simulink model "hbf_fft"  (R2015a)
settings: Solver=ode45  StartTime=0.0  StopTime=240300  RelTol=1e-3
model workspace (MAT data in the model file):
  AD_BP = Simulink.Parameter
  AD_BP.Value = 13
  AD_BP.DataType = 'auto'
  AD_W = Simulink.Parameter
  AD_W.Value = 14
  AD_W.DataType = 'auto'
undefined symbols (not defined in the file or in its folder): a, b
libraries: xbsIndex_r4 x234, dspswit3 x1, commanapbnd3 x1, commseqgen2 x1, dspsigops x1
(part 1 of 2)
settings Model: Creator=scott rogers  LastModifiedBy=scott rogers

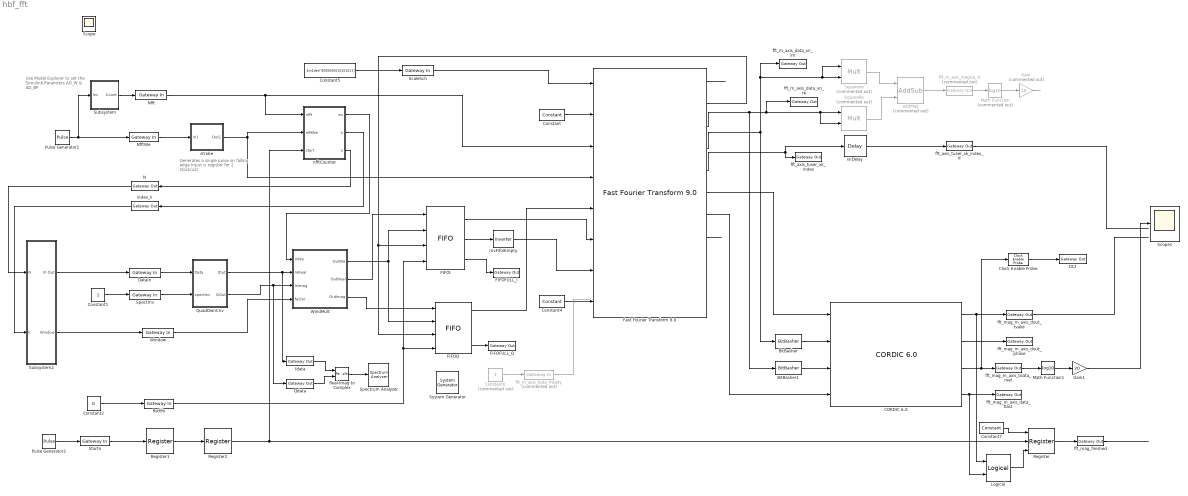
== system hbf_fft ==
  note: Generates a single pulse
      | on falling edge
      | Input is register for 2 Clock(x2)
  note: Use Model Explorer
      | to set the
      | Simulink.Paramters
      | AD_W &  AD_BP
  " System Generator" : xbsIndex_r4/ System Generator  Tag=genX  xilinxfamily=kintex7  part=xc7k160t  speed=-3  package=fbg676  synthesis_tool=Vivado  clock_wrapper=Clock Enables  directory=./netlist  proj_type=Vivado  Synth_file=Vivado Synthesis Defaults  Impl_file=Vivado Implementation Defaults  testbench=off  simulink_period=1  sysclk_period=10  dcm_input_clock_period=10  incr_netlist=off  trim_vbits=Everywhere in SubSystem  dbl_ovrd=According to Block Masks  core_generation=According to Block Masks  run_coregen=off  deprecated_control=off  eval_field=0  block_type=sysgen
  BitBasher : xbsIndex_r4/BitBasher  bitexpr=a={b[15],b[15:0]}  display_expr=off  sr_1=a  arith_type1="Signed  (2's comp)"  bin_pt1=15  sr_2=2  arith_type2=Unsigned  bin_pt2=0  sr_3=3  arith_type3=Unsigned  bin_pt3=0  sr_4=4  arith_type4=Unsigned  bin_pt4=0  dbl_ovrd=off  block_type=bitbasher
  BitBasher1 : xbsIndex_r4/BitBasher  bitexpr=a={b[15],b[15:0]}  display_expr=off  sr_1=a  arith_type1="Signed  (2's comp)"  bin_pt1=15  sr_2=2  arith_type2=Unsigned  bin_pt2=0  sr_3=3  arith_type3=Unsigned  bin_pt3=0  sr_4=4  arith_type4=Unsigned  bin_pt4=0  dbl_ovrd=off  block_type=bitbasher
  CE2 : xbsIndex_r4/Gateway Out  inherit_from_input=off  hdl_port=on  rows=1  columns=1  UseAsDAC=off  DACChannel='1'  interface=None  automatic_assignment=on  address_offset=hex2dec('00')  intf_name=''  intf_description=''  timing_constraint=None  locs_specified=off  LOCs={}  io_standard={}  block_type=gatewayout
  "CORDIC 6.0 " : xbsIndex_r4/CORDIC 6.0   functional_selection=Translate  architectural_configuration=Parallel  pipelining_mode=Maximum  data_format=UnsignedInteger  phase_format=Scaled_Radians  input_width=17  output_width=16  round_mode=Truncate  iterations=0  precision=0  compensation_scaling=No_Scale_Compensation  coarse_rotation=on  aclken=off  aresetn=off  out_tready=off  cartesian_has_tuser=off  cartesian_has_tlast=on  cartesian_tuser_width=1  phase_has_tuser=off  phase_has_tlast=off  phase_tuser_width=1  out_tlast_behv=Null  flow_control=NonBlocking  optimize_goal=Resources  trim_axipin_name=off  simulation_type=hybrid_sim  simulation_model=sysgen:cordic_v6_0  data_path_portlist={'s_axis_cartesian_tdata_imag', 's_axis_cartesian_tdata_real', 's_axis_phase_tdata_phase', 'm_axis_dout_tdata_imag', 'm_axis_dout_tdata_real', 'm_axis_dout_tdata_phase','m_axis_dout_tdata'}  ip_name=CORDIC  ip_version=6.0  dsptool_ready=true  ipcore_usecache=true  ipcore_useipmodelcache=true  wrapper_available=true  port_translation_map={ 'aclken' => 'en', 'aresetn' => 'rst' }  block_type=cordic_v6_0
      settings: infoedit=CORDIC 6.0
  Clock Enable Probe : xbsIndex_r4/Clock Enable Probe  inherit_constraints=on  block_type=ceprobe
      settings: infoedit="Clock enable extractor.  Produces a Boolean output that mirrors the hardware clock enable associated with the input sample rate.<br><br>Hardware notes: in hardware this block costs nothing."
  Constant : xbsIndex_r4/Constant  const=1.0  gui_display_data_type=Fixed-point  arith_type=Unsigned  n_bits=1  bin_pt=0  preci_type=Single  exp_width=8  frac_width=24  explicit_period=off  period=1  equ=P=C  opselect=C  inp2=PCIN>>17  opr=+  inp1=P  carry=CIN  dbl_ovrd=off  block_type=constant
  Constant1 : Constant
  Constant2 : Constant  Value=0
  Constant4 : xbsIndex_r4/Constant  const=0  gui_display_data_type=Boolean  arith_type=Boolean  n_bits=16  bin_pt=14  preci_type=Single  exp_width=8  frac_width=24  explicit_period=off  period=1  equ=P=C  opselect=C  inp2=PCIN>>17  opr=+  inp1=P  carry=CIN  dbl_ovrd=off  block_type=constant
  Constant5 : Constant  Value=bin2dec('0000000010101011')
  Constant6 : Constant  Commented=on
  Constant7 : xbsIndex_r4/Constant  const=1.0  gui_display_data_type=Boolean  arith_type=Boolean  n_bits=1  bin_pt=0  preci_type=Single  exp_width=8  frac_width=24  explicit_period=off  period=1  equ=P=C  opselect=C  inp2=PCIN>>17  opr=+  inp1=P  carry=CIN  dbl_ovrd=off  block_type=constant
  DataIn : xbsIndex_r4/Gateway In  gui_display_data_type=Fixed-point  arith_type="Signed  (2's comp)"  n_bits=AD_W  bin_pt=AD_BP  preci_type=Single  exp_width=8  frac_width=24  rows=1  columns=1  quantization="Round  (unbiased: +/- Inf)"  overflow=Saturate  period=1  UseAsADC=off  ADCChannel='1'  interface=None  automatic_assignment=on  address_offset=hex2dec('00')  intf_name=''  intf_description=''  timing_constraint=None  locs_specified=off  LOCs={}  io_standard={}  inherit_from_input=off  hdl_port=on  dbl_ovrd=off  block_type=gatewayin
  FIFOFULL_I : xbsIndex_r4/Gateway Out  inherit_from_input=off  hdl_port=on  rows=1  columns=1  UseAsDAC=off  DACChannel='1'  interface=None  automatic_assignment=on  address_offset=hex2dec('00')  intf_name=''  intf_description=''  timing_constraint=None  locs_specified=off  LOCs={}  io_standard={}  block_type=gatewayout
  FIFOFULL_Q : xbsIndex_r4/Gateway Out  inherit_from_input=off  hdl_port=on  rows=1  columns=1  UseAsDAC=off  DACChannel='1'  interface=None  automatic_assignment=on  address_offset=hex2dec('00')  intf_name=''  intf_description=''  timing_constraint=None  locs_specified=off  LOCs={}  io_standard={}  block_type=gatewayout
  FIFOI : xbsIndex_r4/FIFO  mem_type=Block RAM  performance_options=Standard_FIFO  embedded_registers=off  depth=16  percent_nbits=2  rst=on  rst_latency=1  en=off  use_dcount=off  use_percent_full_port=off  use_almost_empty=off  almost_empty_thresh=2  use_almost_full=off  almost_full_thresh=14  explicit_period=off  dbl_ovrd=off  block_type=fifo
  FIFOQ : xbsIndex_r4/FIFO  mem_type=Block RAM  performance_options=Standard_FIFO  embedded_registers=off  depth=16  percent_nbits=1  rst=on  rst_latency=1  en=off  use_dcount=off  use_percent_full_port=off  use_almost_empty=off  almost_empty_thresh=2  use_almost_full=off  almost_full_thresh=14  explicit_period=off  dbl_ovrd=off  block_type=fifo
  "Fast Fourier Transform 9.0 " : xbsIndex_r4/Fast Fourier Transform 9.0   transform_length=4096  target_clock_frequency=93  target_data_throughput=50  implementation_options=radix_4_burst_io  run_time_configurable_transform_length=on  phase_factor_width=32  scaling_options=scaled  rounding_modes=truncation  aclken=off  aresetn=off  cyclic_prefix_insertion=off  output_ordering=natural_order  throttle_scheme=realtime  xk_index=on  ovflo=off  trim_axipin_name=off  memory_options_data=block_ram  memory_options_phase_factors=block_ram  number_of_stages_using_block_ram_for_data_and_phase_factors=1  memory_options_reorder=block_ram  memory_options_hybrid=off  complex_mult_type=use_mults_resources  butterfly_type=use_luts  simulation_type=hybrid_sim  simulation_model=sysgen:xfftv9_cmodel  data_path_portlist={ 's_axis_data_tdata', 'm_axis_data_tdata', 'm_axis_status_tdata', 'event_fft_overflow' }  channels=1  input_ordering=natural_order  input_width=16  ip_name=Fast Fourier Transform  ip_version=9.0  dsptool_ready=true  ipcore_usecache=true  ipcore_useipmodelcache=true  wrapper_available=true  port_translation_map={ 'aclken' => 'en', 'aresetn' => 'rst'}  data_format=fixed_point  block_type=xfft_v9_0
  Gain : Gain  Commented=on  Gain=10
  Gain1 : Gain  Gain=20
  Idata : xbsIndex_r4/Gateway Out  inherit_from_input=off  hdl_port=on  rows=1  columns=1  UseAsDAC=off  DACChannel='1'  interface=None  automatic_assignment=on  address_offset=hex2dec('00')  intf_name=''  intf_description=''  timing_constraint=None  locs_specified=off  LOCs={}  io_standard={}  block_type=gatewayout
  InvFifoIEmpty : xbsIndex_r4/Inverter  en=off  latency=0  dbl_ovrd=off  block_type=inv
  Logical : xbsIndex_r4/Logical  logical_function=AND  inputs=2  en=off  latency=1  precision=Full  arith_type=Unsigned  n_bits=16  bin_pt=0  align_bp=on  dbl_ovrd=off  block_type=logical
  Math Function : Math  Commented=on  Operator=log10  SaturateOnIntegerOverflow=on
  Math Function1 : Math  Operator=log10  SaturateOnIntegerOverflow=on
  N : xbsIndex_r4/Gateway Out  inherit_from_input=off  hdl_port=on  rows=1  columns=1  UseAsDAC=off  DACChannel='1'  interface=None  automatic_assignment=on  address_offset=hex2dec('00')  intf_name=''  intf_description=''  timing_constraint=None  locs_specified=off  LOCs={}  io_standard={}  block_type=gatewayout
  Nfft : xbsIndex_r4/Gateway In  gui_display_data_type=Fixed-point  arith_type=Unsigned  n_bits=5  bin_pt=0  preci_type=Single  exp_width=8  frac_width=24  rows=1  columns=1  quantization="Round  (unbiased: +/- Inf)"  overflow=Wrap  period=2  UseAsADC=off  ADCChannel='1'  interface=None  automatic_assignment=on  address_offset=hex2dec('00')  intf_name=''  intf_description=''  timing_constraint=None  locs_specified=off  LOCs={}  io_standard={}  inherit_from_input=off  hdl_port=on  dbl_ovrd=off  block_type=gatewayin
  NfftWe : xbsIndex_r4/Gateway In  gui_display_data_type=Boolean  arith_type=Boolean  n_bits=16  bin_pt=14  preci_type=Single  exp_width=8  frac_width=24  rows=1  columns=1  quantization="Round  (unbiased: +/- Inf)"  overflow=Saturate  period=2  UseAsADC=off  ADCChannel='1'  interface=None  automatic_assignment=on  address_offset=hex2dec('00')  intf_name=''  intf_description=''  timing_constraint=None  locs_specified=off  LOCs={}  io_standard={}  inherit_from_input=off  hdl_port=on  dbl_ovrd=off  block_type=gatewayin
  Pulse Generator1 : DiscretePulseGenerator  Period=30000  PulseWidth=8  PhaseDelay=10
  Pulse Generator2 : DiscretePulseGenerator  Period=30000  PulseWidth=21  PhaseDelay=38
  Qdata : xbsIndex_r4/Gateway Out  inherit_from_input=off  hdl_port=on  rows=1  columns=1  UseAsDAC=off  DACChannel='1'  interface=None  automatic_assignment=on  address_offset=hex2dec('00')  intf_name=''  intf_description=''  timing_constraint=None  locs_specified=off  LOCs={}  io_standard={}  block_type=gatewayout
  QuadDwnCnv : Subsystem
  Real-Imag to Complex : RealImagToComplex
  Register : xbsIndex_r4/Register  init=0  rst=on  en=on  dbl_ovrd=off  block_type=register
  Register1 : xbsIndex_r4/Register  init=0  rst=off  en=off  dbl_ovrd=off  block_type=register
  Register2 : xbsIndex_r4/Register  init=0  rst=off  en=off  dbl_ovrd=off  block_type=register
  Rstfifo : xbsIndex_r4/Gateway In  gui_display_data_type=Boolean  arith_type=Boolean  n_bits=16  bin_pt=14  preci_type=Single  exp_width=8  frac_width=24  rows=1  columns=1  quantization="Round  (unbiased: +/- Inf)"  overflow=Saturate  period=2  UseAsADC=off  ADCChannel='1'  interface=None  automatic_assignment=on  address_offset=hex2dec('00')  intf_name=''  intf_description=''  timing_constraint=None  locs_specified=off  LOCs={}  io_standard={}  inherit_from_input=off  hdl_port=on  dbl_ovrd=off  block_type=gatewayin
  ScaleSch : xbsIndex_r4/Gateway In  gui_display_data_type=Fixed-point  arith_type=Unsigned  n_bits=12  bin_pt=0  preci_type=Single  exp_width=8  frac_width=24  rows=1  columns=1  quantization="Round  (unbiased: +/- Inf)"  overflow=Wrap  period=2  UseAsADC=off  ADCChannel='1'  interface=None  automatic_assignment=on  address_offset=hex2dec('00')  intf_name=''  intf_description=''  timing_constraint=None  locs_specified=off  LOCs={}  io_standard={}  inherit_from_input=off  hdl_port=on  dbl_ovrd=off  block_type=gatewayin
  Scope1 : Scope
      settings: TimeRange=200000  YMin=-51.8234  YMax=-51.8234  MaxDataPoints=15000
  SpectInv : xbsIndex_r4/Gateway In  gui_display_data_type=Fixed-point  arith_type=Unsigned  n_bits=1  bin_pt=0  preci_type=Single  exp_width=8  frac_width=24  rows=1  columns=1  quantization="Round  (unbiased: +/- Inf)"  overflow=Wrap  period=2  UseAsADC=off  ADCChannel='1'  interface=None  automatic_assignment=on  address_offset=hex2dec('00')  intf_name=''  intf_description=''  timing_constraint=None  locs_specified=off  LOCs={}  io_standard={}  inherit_from_input=off  hdl_port=on  dbl_ovrd=off  block_type=gatewayin
  Spectrum Analyzer : SpectrumAnalyzer
  SquareIm : xbsIndex_r4/Mult  Commented=on  precision=Full  arith_type="Signed  (2's comp)"  n_bits=17  bin_pt=15  quantization=Truncate  overflow=Wrap  en=off  latency=3  use_behavioral_HDL=off  opt=Speed  use_embedded=on  optimum_pipeline=off  pipeline=on  dbl_ovrd=off  use_rpm=on  placement_style=Triangular  block_type=mult
  SquareRe : xbsIndex_r4/Mult  Commented=on  precision=Full  arith_type="Signed  (2's comp)"  n_bits=17  bin_pt=15  quantization=Truncate  overflow=Wrap  en=off  latency=3  use_behavioral_HDL=off  opt=Speed  use_embedded=on  optimum_pipeline=off  pipeline=on  dbl_ovrd=off  use_rpm=on  placement_style=Triangular  block_type=mult
  Startn : xbsIndex_r4/Gateway In  gui_display_data_type=Boolean  arith_type=Boolean  n_bits=16  bin_pt=14  preci_type=Single  exp_width=8  frac_width=24  rows=1  columns=1  quantization="Round  (unbiased: +/- Inf)"  overflow=Saturate  period=2  UseAsADC=off  ADCChannel='1'  interface=None  automatic_assignment=on  address_offset=hex2dec('00')  intf_name=''  intf_description=''  timing_constraint=None  locs_specified=off  LOCs={}  io_standard={}  inherit_from_input=off  hdl_port=on  dbl_ovrd=off  block_type=gatewayin
  Subsystem : Subsystem
  Subsystem2 : Subsystem
  WindMult : Subsystem
  Window : xbsIndex_r4/Gateway In  gui_display_data_type=Fixed-point  arith_type=Unsigned  n_bits=16  bin_pt=14  preci_type=Single  exp_width=8  frac_width=24  rows=1  columns=1  quantization="Round  (unbiased: +/- Inf)"  overflow=Wrap  period=2  UseAsADC=off  ADCChannel='1'  interface=None  automatic_assignment=on  address_offset=hex2dec('00')  intf_name=''  intf_description=''  timing_constraint=None  locs_specified=off  LOCs={}  io_standard={}  inherit_from_input=off  hdl_port=on  dbl_ovrd=off  block_type=gatewayin
  addMag : xbsIndex_r4/AddSub  Commented=on  mode=Addition  use_carryin=off  use_carryout=off  en=off  latency=1  precision=Full  arith_type=Unsigned  n_bits=16  bin_pt=14  quantization=Truncate  overflow=Wrap  use_behavioral_HDL=off  hw_selection=Fabric  pipelined=off  dbl_ovrd=off  block_type=addsub
  fft_axis_tuser_xk_index : xbsIndex_r4/Gateway Out  inherit_from_input=off  hdl_port=off  rows=1  columns=1  UseAsDAC=off  DACChannel='1'  interface=None  automatic_assignment=on  address_offset=hex2dec('00')  intf_name=''  intf_description=''  timing_constraint=None  locs_specified=off  LOCs={}  io_standard={}  block_type=gatewayout
  fft_axis_tuser_xk_index_d : xbsIndex_r4/Gateway Out  inherit_from_input=off  hdl_port=on  rows=1  columns=1  UseAsDAC=off  DACChannel='1'  interface=None  automatic_assignment=on  address_offset=hex2dec('00')  intf_name=''  intf_description=''  timing_constraint=None  locs_specified=off  LOCs={}  io_standard={}  block_type=gatewayout
  fft_m_axis_data_tready : xbsIndex_r4/Gateway In  Commented=on  gui_display_data_type=Boolean  arith_type=Boolean  n_bits=16  bin_pt=14  preci_type=Single  exp_width=8  frac_width=24  rows=1  columns=1  quantization="Round  (unbiased: +/- Inf)"  overflow=Saturate  period=2  UseAsADC=off  ADCChannel='1'  interface=None  automatic_assignment=on  address_offset=hex2dec('00')  intf_name=''  intf_description=''  timing_constraint=None  locs_specified=off  LOCs={}  io_standard={}  inherit_from_input=off  hdl_port=on  dbl_ovrd=off  block_type=gatewayin
  fft_m_axis_data_xn_im : xbsIndex_r4/Gateway Out  inherit_from_input=off  hdl_port=off  rows=1  columns=1  UseAsDAC=off  DACChannel='1'  interface=None  automatic_assignment=on  address_offset=hex2dec('00')  intf_name=''  intf_description=''  timing_constraint=None  locs_specified=off  LOCs={}  io_standard={}  block_type=gatewayout
  fft_m_axis_data_xn_re : xbsIndex_r4/Gateway Out  inherit_from_input=off  hdl_port=off  rows=1  columns=1  UseAsDAC=off  DACChannel='1'  interface=None  automatic_assignment=on  address_offset=hex2dec('00')  intf_name=''  intf_description=''  timing_constraint=None  locs_specified=off  LOCs={}  io_standard={}  block_type=gatewayout
  fft_m_axis_magSq_d : xbsIndex_r4/Gateway Out  Commented=on  inherit_from_input=off  hdl_port=on  rows=1  columns=1  UseAsDAC=off  DACChannel='1'  interface=None  automatic_assignment=on  address_offset=hex2dec('00')  intf_name=''  intf_description=''  timing_constraint=None  locs_specified=off  LOCs={}  io_standard={}  block_type=gatewayout
  fft_mag_finished : xbsIndex_r4/Gateway Out  inherit_from_input=off  hdl_port=on  rows=1  columns=1  UseAsDAC=off  DACChannel='1'  interface=None  automatic_assignment=on  address_offset=hex2dec('00')  intf_name=''  intf_description=''  timing_constraint=None  locs_specified=off  LOCs={}  io_standard={}  block_type=gatewayout
  fft_mag_m_axis_data_tlast : xbsIndex_r4/Gateway Out  inherit_from_input=off  hdl_port=on  rows=1  columns=1  UseAsDAC=off  DACChannel='1'  interface=None  automatic_assignment=on  address_offset=hex2dec('00')  intf_name=''  intf_description=''  timing_constraint=None  locs_specified=off  LOCs={}  io_standard={}  block_type=gatewayout
  fft_mag_m_axis_dout_phase : xbsIndex_r4/Gateway Out  inherit_from_input=off  hdl_port=off  rows=1  columns=1  UseAsDAC=off  DACChannel='1'  interface=None  automatic_assignment=on  address_offset=hex2dec('00')  intf_name=''  intf_description=''  timing_constraint=None  locs_specified=off  LOCs={}  io_standard={}  block_type=gatewayout
  fft_mag_m_axis_dout_tvalid : xbsIndex_r4/Gateway Out  inherit_from_input=off  hdl_port=on  rows=1  columns=1  UseAsDAC=off  DACChannel='1'  interface=None  automatic_assignment=on  address_offset=hex2dec('00')  intf_name=''  intf_description=''  timing_constraint=None  locs_specified=off  LOCs={}  io_standard={}  block_type=gatewayout
  fft_mag_m_axis_tdata_real : xbsIndex_r4/Gateway Out  inherit_from_input=off  hdl_port=on  rows=1  columns=1  UseAsDAC=off  DACChannel='1'  interface=None  automatic_assignment=on  address_offset=hex2dec('00')  intf_name=''  intf_description=''  timing_constraint=None  locs_specified=off  LOCs={}  io_standard={}  block_type=gatewayout
  index_k : xbsIndex_r4/Gateway Out  inherit_from_input=off  hdl_port=on  rows=1  columns=1  UseAsDAC=off  DACChannel='1'  interface=None  automatic_assignment=on  address_offset=hex2dec('00')  intf_name=''  intf_description=''  timing_constraint=None  locs_specified=off  LOCs={}  io_standard={}  block_type=gatewayout
  nfftCounter : Subsystem
  strobe : Subsystem
  xnDelay : xbsIndex_r4/Delay  rst=off  infoeditControl=Selection of Reset will increase slice count due to use of real FFs and instead of SRLs  en=off  latency=20  reg_retiming=on  dbl_ovrd=off  block_type=delay
  Scope : Scope
  wires:
  FIFOI/2 -> InvFifoIEmpty/1
  InvFifoIEmpty/1 -> "Fast Fourier Transform 9.0 "/7
  FIFOI/1 -> "Fast Fourier Transform 9.0 "/6
  FIFOQ/1 -> "Fast Fourier Transform 9.0 "/5
  Nfft/1 -> "Fast Fourier Transform 9.0 "/3, nfftCounter/1(nfft)
  Constant/1 -> "Fast Fourier Transform 9.0 "/2
  Startn/1 -> Register1/1
  "Fast Fourier Transform 9.0 "/5 -> fft_axis_tuser_xk_index/1, xnDelay/1
  "Fast Fourier Transform 9.0 "/4 -> BitBasher/1, SquareIm/2, SquareIm/1, fft_m_axis_data_xn_im/1
  Pulse Generator2/1 -> Startn/1
  "Fast Fourier Transform 9.0 "/2 -> FIFOQ/3, FIFOI/3
  FIFOQ/3 -> FIFOFULL_Q/1
  FIFOI/3 -> FIFOFULL_I/1
  Constant4/1 -> "Fast Fourier Transform 9.0 "/8
  nfftCounter/1(en) -> WindMult/1(InWe)
  DataIn/1 -> QuadDwnCnv/1(Data)
  SquareIm/1 -> addMag/1
  SquareRe/1 -> addMag/2
  Pulse Generator1/1 -> NfftWe/1, Subsystem/1(Inc)
  Idata/1 -> Real-Imag to Complex/1
  Qdata/1 -> Real-Imag to Complex/2
  addMag/1 -> fft_m_axis_magSq_d/1
  SpectInv/1 -> QuadDwnCnv/2(spectInv)
  Constant1/1 -> SpectInv/1
  fft_m_axis_magSq_d/1 -> Math Function/1
  Math Function/1 -> Gain/1
  Gain/1 -> ?
  xnDelay/1 -> fft_axis_tuser_xk_index_d/1
  Constant2/1 -> Rstfifo/1
  Rstfifo/1 -> FIFOQ/4, FIFOI/4
  Constant6/1 -> fft_m_axis_data_tready/1
  fft_mag_m_axis_tdata_real/1 -> Math Function1/1
  Math Function1/1 -> Gain1/1
  Gain1/1 -> Scope1/1
  BitBasher/1 -> "CORDIC 6.0 "/2
  BitBasher1/1 -> "CORDIC 6.0 "/3
  fft_mag_m_axis_dout_tvalid/1 -> ?
  "CORDIC 6.0 "/1 -> Logical/1, fft_mag_m_axis_dout_tvalid/1
  "CORDIC 6.0 "/4 -> Logical/2, fft_mag_m_axis_data_tlast/1
  "Fast Fourier Transform 9.0 "/7 -> "CORDIC 6.0 "/4
  fft_axis_tuser_xk_index_d/1 -> ?
  "CORDIC 6.0 "/2 -> fft_mag_m_axis_dout_phase/1
  Constant7/1 -> Register/1
  Register/1 -> fft_mag_finished/1
  fft_mag_finished/1 -> ?
  strobe/1(Out1) -> "Fast Fourier Transform 9.0 "/4, nfftCounter/2(nfftWe)
  QuadDwnCnv/2(QOut) -> Qdata/1, WindMult/3(InImag)
  QuadDwnCnv/1(IOut) -> Idata/1, WindMult/2(inReal)
  nfftCounter/2(k) -> index_k/1
  Window/1 -> WindMult/4(factor)
  WindMult/2(OutReal) -> FIFOI/1
  WindMult/3(OutImag) -> FIFOQ/1
  WindMult/1(OutWe) -> FIFOQ/2, FIFOI/2
  nfftCounter/3(n) -> N/1
  Register1/1 -> Register2/1
  "Fast Fourier Transform 9.0 "/3 -> BitBasher1/1, fft_m_axis_data_xn_re/1, SquareRe/2, SquareRe/1
  Register2/1 -> Register/2, nfftCounter/3(start)
  Subsystem/1(Count) -> Nfft/1
  NfftWe/1 -> strobe/1(In1)
  N/1 -> Subsystem2/1(N)
  index_k/1 -> Subsystem2/2(k)
  Subsystem2/1(IF Out) -> DataIn/1
  Subsystem2/2(Window) -> Window/1
  "Fast Fourier Transform 9.0 "/6 -> "CORDIC 6.0 "/1
  "CORDIC 6.0 "/3 -> Clock Enable Probe/1, fft_mag_m_axis_tdata_real/1
  fft_m_axis_data_tready/1 -> ?
  "Fast Fourier Transform 9.0 "/8 -> ?
  Real-Imag to Complex/1 -> Spectrum Analyzer/1
  ScaleSch/1 -> "Fast Fourier Transform 9.0 "/1
  Constant5/1 -> ScaleSch/1
  "Fast Fourier Transform 9.0 "/1 -> ?
  Logical/1 -> Register/3
  Clock Enable Probe/1 -> CE2/1

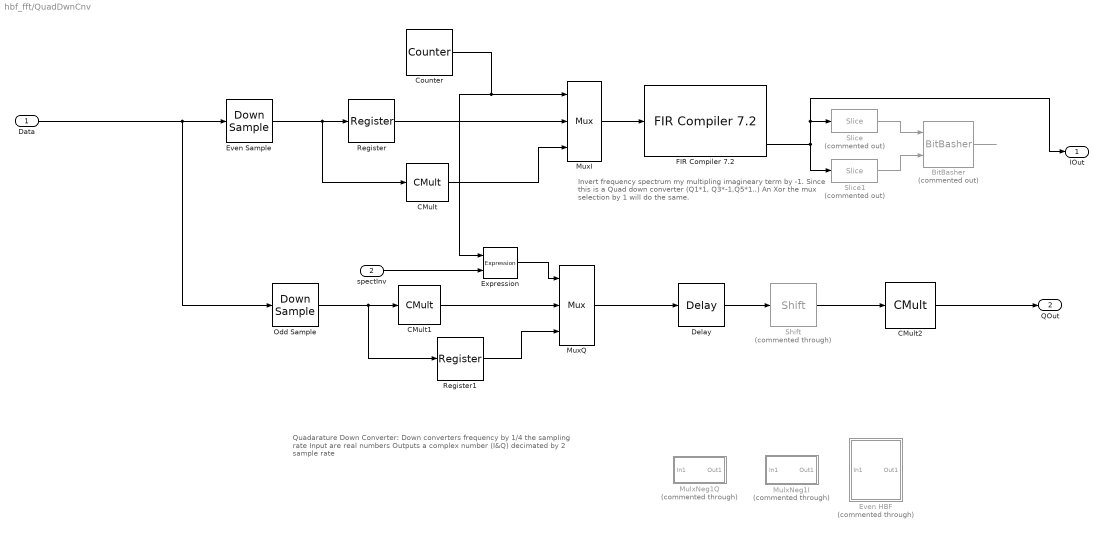
== system hbf_fft/QuadDwnCnv ==
  note: Invert frequency spectrum my multipling imagineary term by -1.
      | Since this is a Quad down converter (Q1*1, Q3*-1,Q5*1..)
      | An Xor the mux selection by 1 will do the same.
  note: Quadarature Down Converter:
      | Down converters frequency by 1/4 the sampling rate
      | Input are real numbers
      | Outputs a complex number (I&Q) decimated by 2 sample rate
  Data : Inport
  spectInv : Inport  Port=2
  BitBasher : xbsIndex_r4/BitBasher  Commented=on  bitexpr=a={b,c}  display_expr=off  sr_1=a  arith_type1="Signed  (2's comp)"  bin_pt1=13  sr_2=2  arith_type2=Unsigned  bin_pt2=0  sr_3=3  arith_type3=Unsigned  bin_pt3=0  sr_4=4  arith_type4=Unsigned  bin_pt4=0  dbl_ovrd=off  block_type=bitbasher
  CMult : xbsIndex_r4/CMult  const=-1  gui_display_data_type=Fixed-point  const_n_bits=14  const_bin_pt=13  float_type=Single  exp_bits=8  fraction_bits=24  en=off  latency=1  precision=User Defined  arith_type="Signed  (2's comp)"  n_bits=14  bin_pt=13  quantization=Truncate  overflow=Saturate  use_behavioral_HDL=off  mem_type=Distributed RAM  pipeline=off  dbl_ovrd=off  block_type=cmult
  CMult1 : xbsIndex_r4/CMult  const=-1  gui_display_data_type=Fixed-point  const_n_bits=14  const_bin_pt=13  float_type=Single  exp_bits=8  fraction_bits=24  en=off  latency=1  precision=User Defined  arith_type="Signed  (2's comp)"  n_bits=14  bin_pt=13  quantization=Truncate  overflow=Saturate  use_behavioral_HDL=off  mem_type=Distributed RAM  pipeline=off  dbl_ovrd=off  block_type=cmult
  CMult2 : xbsIndex_r4/CMult  const=.5  gui_display_data_type=Fixed-point  const_n_bits=16  const_bin_pt=14  float_type=Single  exp_bits=8  fraction_bits=24  en=off  latency=1  precision=User Defined  arith_type="Signed  (2's comp)"  n_bits=16  bin_pt=14  quantization=Truncate  overflow=Wrap  use_behavioral_HDL=off  mem_type=Distributed RAM  pipeline=off  dbl_ovrd=off  block_type=cmult
  Counter : xbsIndex_r4/Counter  cnt_type=Count Limited  cnt_to=1  operation=Up  start_count=0  cnt_by_val=1  arith_type=Unsigned  n_bits=1  bin_pt=0  load_pin=off  rst=off  en=off  explicit_period=on  period=2  use_behavioral_HDL=off  implementation=Fabric  dbl_ovrd=off  block_type=counter
  Delay : xbsIndex_r4/Delay  rst=off  infoeditControl=Selection of Reset will increase slice count due to use of real FFs and instead of SRLs  en=off  latency=17  reg_retiming=off  dbl_ovrd=off  block_type=delay
  Even HBF : Subsystem  Commented=through  mask{coe=|, numbits=16, binarypoint=16}
      mask coe=|
      | [5.78745247606902e-07	-6.34583335209700e-06	3.11100665493994e-05	-9.81618504431095e-05	0.000251198104263337	-0.000560678336657476	0.00113068456439032	-0.00210596116830266	0.00368000288358338	-0.00610797832934512	0.00973476334993138	-0.0150640153636479	0.0229388203755087	-0.0350608263163152	0.0557915831460557	-0.101197280248630	0.316642817526843
      | ]
      mask prompts: coe "Coefficent"; numbits "Number of Bits"; binarypoint "Binary Point"
  Even Sample : xbsIndex_r4/Down Sample  sample_ratio=2  sample_phase=First Value of Frame  en=off  rst=off  latency=1  dbl_ovrd=off  block_type=dsamp
  Expression : xbsIndex_r4/Expression  expression=a ^ b  align_bp=on  en=off  latency=0  precision=Full  arith_type=Unsigned  n_bits=16  bin_pt=0  dbl_ovrd=off  block_type=expr
  "FIR Compiler 7.2 " : xbsIndex_r4/FIR Compiler 7.2   coefficientvector=[0.00115083621567666,-0.00274368371137841,0.00575557363771786,-0.0107205402010719,0.0185625473110580,-0.0310523194554332,0.0525318906465399,-0.0990035964397264,0.315519291996618,0.315519291996618,-0.0990035964397264,0.0525318906465399,-0.0310523194554332,0.0185625473110580,-0.0107205402010719,0.00575557363771786,-0.00274368371137841,0.00115083621567666]  coefficient_sets=1  coefficient_reload=off  filter_type=Single_Rate  rate_change_type=Integer  interpolation_rate=1  decimation_rate=1  zero_pack_factor=1  channel_sequence=Basic  number_channels=1  pattern_list='P4-0,P4-1,P4-2,P4-3,P4-4'  number_paths=1  ratespecification=Maximum_Possible  sampleperiod=2  hardwareoversamplingrate=1  coefficient_sign=Signed  quantization=Quantize_Only  coefficient_width=16  bestprecision=on  coefficient_fractional_bits=16  coefficient_structure=Inferred  output_rounding_mode=Truncate_LSBs  output_width=19  filter_architecture=Systolic_Multiply_Accumulate  optimization_goal=Area  optimization_list='None'  data_buffer_type=Automatic  coefficient_buffer_type=Automatic  input_buffer_type=Automatic  output_buffer_type=Automatic  preference_for_other_storage=Automatic  multi_column_support=Automatic  columnconfig='9'  inter_column_pipe_length=4  data_has_tlast=Not_Required  m_data_has_tready=off  s_data_has_fifo=off  s_data_has_tuser=Not_Required  m_data_has_tuser=Not_Required  s_config_sync_mode=On_Vector  s_config_method=Single  num_reload_slots=1  has_aclken=off  has_aresetn=off  infoeditControl=ARESETn must be asserted for a minimum of 2 cycles  reset_data_vector=on  trim_axipin_name=on  simulation_type=hybrid_sim  simulation_model=sysgen:xfirv7_2_cmodel  data_path_portlist={ 's_axis_data_tdata', 'm_axis_data_tdata' }  passband_min=0.0  passband_max=0.5  stopband_min=0.5  stopband_max=1.0  filter_selection=1  gui_behaviour='Sysgen_GUI'  data_sign=Signed  data_width=16  data_fractional_bits=0  data_tuser_width=1  wrapper_available=true  ip_wrap_arbitrary_binary_point=true  ip_name=FIR Compiler  ip_version=7.2  dsptool_ready=true  ipcore_usecache=true  ipcore_useipmodelcache=true  port_translation_map={ 'aclken' => 'en', 'aresetn' => 'rst' }  run_core_at_system_period=true  ipcore_xco_need_fpga_part=true  block_type=fir_compiler_v7_2
      settings: infoedit=Maximum Possible : Maximizes oversampling rate. Abstracted input handshake (no s_data_tvalid) and automatic rate propagation.<br>Hardware Oversampling Rate : Specifies oversampling rate relative to the input sample period. Abstracted input handshake (no s_data_tvalid) and automatic rate propagation.<br>Input/Output Sample Period : Specifies absolute oversampling rate. No input handshake abstraction (exposes s_data_tvalid) and no rate propagation.
  MulxNeg1I : Subsystem  Commented=through
  MulxNeg1Q : Subsystem  Commented=through
  MuxI : xbsIndex_r4/Mux  inputs=2  en=off  latency=1  precision=Full  arith_type=Unsigned  n_bits=16  bin_pt=14  quantization=Truncate  overflow=Wrap  dbl_ovrd=off  block_type=mux
  MuxQ : xbsIndex_r4/Mux  inputs=2  en=off  latency=1  precision=Full  arith_type=Unsigned  n_bits=16  bin_pt=14  quantization=Truncate  overflow=Wrap  dbl_ovrd=off  block_type=mux
  Odd Sample : xbsIndex_r4/Down Sample  sample_ratio=2  sample_phase="Last Value of Frame  (most efficient)"  en=off  rst=off  latency=1  dbl_ovrd=off  block_type=dsamp
  Register : xbsIndex_r4/Register  init=0  rst=off  en=off  dbl_ovrd=off  block_type=register
  Register1 : xbsIndex_r4/Register  init=0  rst=off  en=off  dbl_ovrd=off  block_type=register
  Shift : xbsIndex_r4/Shift  Commented=through  shift_dir=Right  shift_bits=1  en=off  latency=1  precision=Full  arith_type="Signed  (2's comp)"  n_bits=15  bin_pt=14  quantization=Truncate  overflow=Wrap  dbl_ovrd=off  block_type=shift
  Slice : xbsIndex_r4/Slice  Commented=on  nbits=1  boolean_output=off  mode=Upper Bit Location + Width  bit1=0  base1=MSB of Input  bit0=-13  base0=Binary Point of Input  dbl_ovrd=off  block_type=slice
  Slice1 : xbsIndex_r4/Slice  Commented=on  nbits=13  boolean_output=off  mode=Two Bit Locations  bit1=-1  base1=Binary Point of Input  bit0=-13  base0=Binary Point of Input  dbl_ovrd=off  block_type=slice
  IOut : Outport
  QOut : Outport  Port=2
  wires:
  Even Sample/1 -> CMult/1, Register/1
  CMult1/1 -> MuxQ/2
  Counter/1 -> MuxI/1, Expression/1
  Odd Sample/1 -> CMult1/1, Register1/1
  Register/1 -> MuxI/2
  Register1/1 -> MuxQ/3
  Expression/1 -> MuxQ/1
  spectInv/1 -> Expression/2
  Data/1 -> Odd Sample/1, Even Sample/1
  Delay/1 -> Shift/1
  MuxI/1 -> "FIR Compiler 7.2 "/1
  MuxQ/1 -> Delay/1
  Shift/1 -> CMult2/1
  "FIR Compiler 7.2 "/3 -> Slice1/1, IOut/1, Slice/1
  Slice/1 -> BitBasher/1
  BitBasher/1 -> ?
  Slice1/1 -> BitBasher/2
  CMult/1 -> MuxI/3
  CMult2/1 -> QOut/1

== system hbf_fft/Subsystem ==
  Inc : Inport
  Constant : Constant  Value=10
  Counter : dspswit3/Counter  Direction=Up  CountEvent=Falling edge  CounterSize=User defined  MaxCount=1  InitialCount=0  Output=Count  HitValue=32  ResetInput=off  SamplesPerFrame=1  Ts=1  CntDtype=double  HitDtype=Logical
  Manual Switch : ManualSwitch  CurrentSetting=0
  Sum : Sum  Inputs=|++
  Count : Outport
  wires:
  Inc/1 -> Counter/1
  Counter/1 -> Sum/1
  Constant/1 -> Manual Switch/2, Sum/2
  Sum/1 -> Manual Switch/1
  Manual Switch/1 -> Count/1

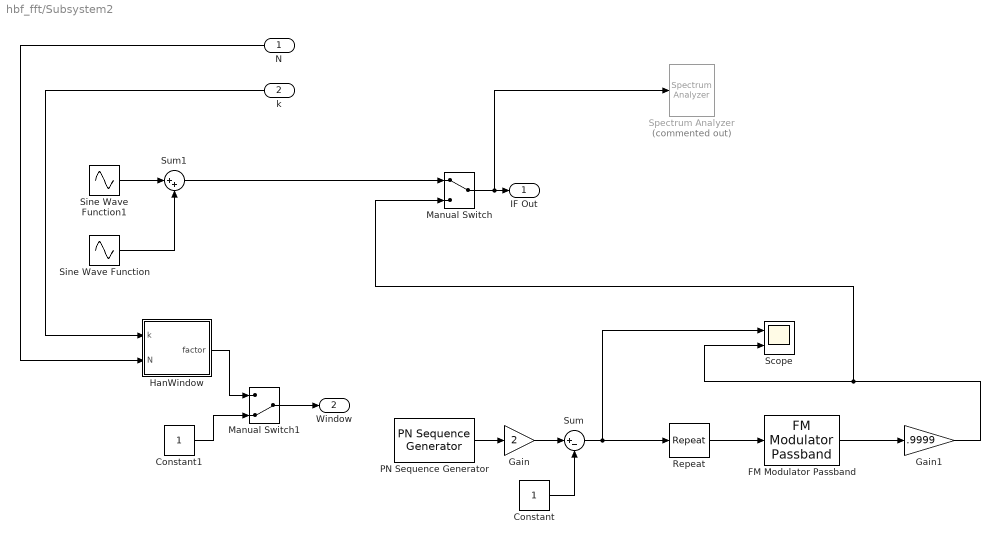
== system hbf_fft/Subsystem2 ==
  N : Inport
  k : Inport  Port=2
  Constant : Constant
  Constant1 : Constant
  FM Modulator Passband : commanapbnd3/FM Modulator Passband  Fc=76/93.3333  Ph=0  Kc=1.81/93.3333
  Gain : Gain  Gain=2
  Gain1 : Gain  Gain=.9999
  HanWindow : Subsystem
  Manual Switch : ManualSwitch
  Manual Switch1 : ManualSwitch  CurrentSetting=0
  PN Sequence Generator : commseqgen2/PN Sequence Generator  poly=[1 0 0 0 0 1 1]  ini_sta=[0 0 0 0 0 1]  outBitMaskSource=Dialog parameter  shift=0  outVarSiz=off  maxOutSizeMode=Dialog parameter  maxOutSize=[10 1]  Ts=18  frameBased=off  sampPerFrame=1  reset=off  bitPackedOutputs=off  outDataType=double  numPackedBits=8  bitPackDataSigned=off  bitPackedOutDType=double
  Repeat : dspsigops/Repeat  N=18  RateOptions=Allow multirate processing  ic=0  mode=Unused parameter value
  Scope : Scope  NumInputPorts=2
      settings: YMin=-5~-5  YMax=5~5  SaveName=ScopeData2
  Sine Wave Function : Sin  Amplitude=.9  Frequency=75.5/93.3333*2*pi  Phase=pi/2*.3  SampleTime=1
  Sine Wave Function1 : Sin  Amplitude=.0000  Frequency=68/93.3333*2*pi  Phase=.1*pi  Samples=1/(70/93)  SampleTime=1
  Spectrum Analyzer : SpectrumAnalyzer  Commented=on
  Sum : Sum  Inputs=|+-
  Sum1 : Sum  Inputs=|++
  IF Out : Outport
  Window : Outport  Port=2
  wires:
  N/1 -> HanWindow/2(N)
  PN Sequence Generator/1 -> Gain/1
  Gain/1 -> Sum/1
  Constant/1 -> Sum/2
  FM Modulator Passband/1 -> Gain1/1
  Sum/1 -> Repeat/1, Scope/1
  Sine Wave Function/1 -> Sum1/2
  Sine Wave Function1/1 -> Sum1/1
  Sum1/1 -> Manual Switch/1
  Manual Switch/1 -> Spectrum Analyzer/1, IF Out/1
  Constant1/1 -> Manual Switch1/2
  Manual Switch1/1 -> Window/1
  k/1 -> HanWindow/1(k)
  HanWindow/1(factor) -> Manual Switch1/1
  Repeat/1 -> FM Modulator Passband/1
  Gain1/1 -> Manual Switch/2, Scope/2

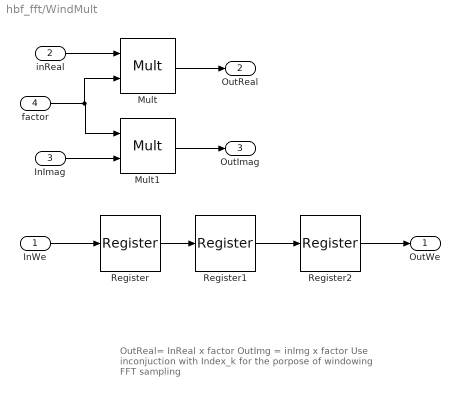
== system hbf_fft/WindMult ==
  note: OutReal= InReal x factor
      | OutImg = inImg x factor
      | Use inconjuction with Index_k
      | for the porpose of windowing
      | FFT sampling
  InWe : Inport
  inReal : Inport  Port=2
  InImag : Inport  Port=3
  factor : Inport  Port=4
  Mult : xbsIndex_r4/Mult  precision=User Defined  arith_type="Signed  (2's comp)"  n_bits=18  bin_pt=17  quantization=Truncate  overflow=Wrap  en=off  latency=3  use_behavioral_HDL=off  opt=Speed  use_embedded=on  optimum_pipeline=off  pipeline=on  dbl_ovrd=off  use_rpm=on  placement_style=Triangular  block_type=mult
  Mult1 : xbsIndex_r4/Mult  precision=User Defined  arith_type="Signed  (2's comp)"  n_bits=18  bin_pt=17  quantization=Truncate  overflow=Wrap  en=off  latency=3  use_behavioral_HDL=off  opt=Speed  use_embedded=on  optimum_pipeline=off  pipeline=on  dbl_ovrd=off  use_rpm=on  placement_style=Triangular  block_type=mult
  Register : xbsIndex_r4/Register  init=0  rst=off  en=off  dbl_ovrd=off  block_type=register
  Register1 : xbsIndex_r4/Register  init=0  rst=off  en=off  dbl_ovrd=off  block_type=register
  Register2 : xbsIndex_r4/Register  init=0  rst=off  en=off  dbl_ovrd=off  block_type=register
  OutWe : Outport
  OutReal : Outport  Port=2
  OutImag : Outport  Port=3
  wires:
  Mult1/1 -> OutImag/1
  factor/1 -> Mult/2, Mult1/1
  Mult/1 -> OutReal/1
  InImag/1 -> Mult1/2
  inReal/1 -> Mult/1
  InWe/1 -> Register/1
  Register/1 -> Register1/1
  Register1/1 -> Register2/1
  Register2/1 -> OutWe/1

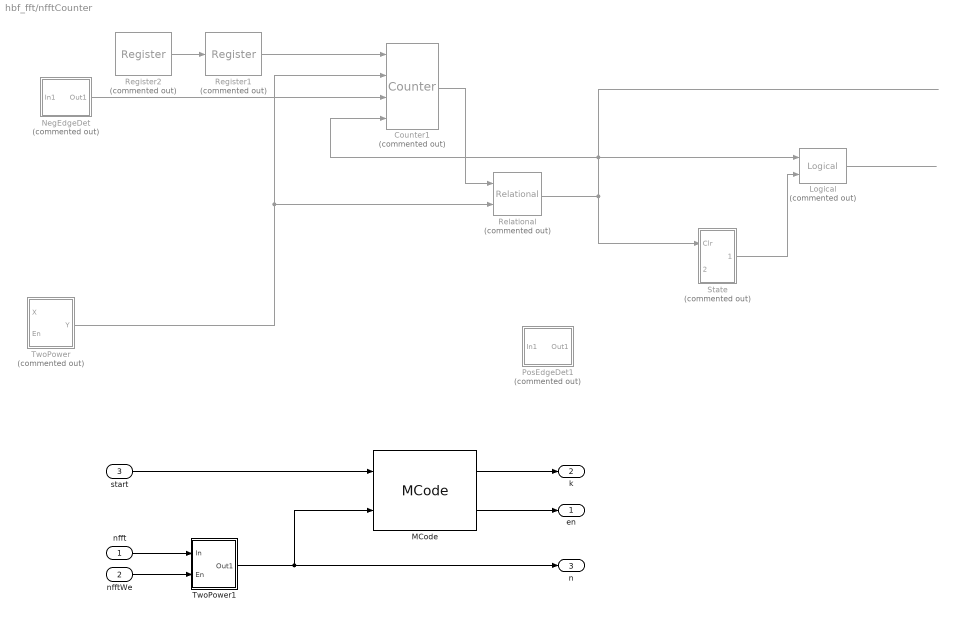
== system hbf_fft/nfftCounter ==
  nfft : Inport
  nfftWe : Inport  Port=2
  start : Inport  Port=3
  Counter1 : xbsIndex_r4/Counter  Commented=on  cnt_type=Free Running  cnt_to=Inf  operation=Up  start_count=0  cnt_by_val=1  arith_type=Unsigned  n_bits=13  bin_pt=0  load_pin=on  rst=on  en=on  explicit_period=on  period=2  use_behavioral_HDL=off  implementation=Fabric  dbl_ovrd=off  block_type=counter
  Logical : xbsIndex_r4/Logical  Commented=on  logical_function=AND  inputs=2  en=off  latency=0  precision=Full  arith_type=Unsigned  n_bits=16  bin_pt=0  align_bp=on  dbl_ovrd=off  block_type=logical
  MCode : xbsIndex_r4/MCode  mfname=kIndexCounter  explicit_period=off  period=1  inputsTable={'boundInpExpr'=>['',''],'inputs'=>['x','y']}  outputsTable={'outputs'=>['z'],'suppressOut'=>['off']}  enable_stdout=off  enable_debug=off  suppress_output=on  defparams={}  hide_port_list={}  dbl_ovrd=off  block_type=mcode
  NegEdgeDet : Subsystem  Commented=on
  PosEdgeDet1 : Subsystem  Commented=on
  Register1 : xbsIndex_r4/Register  Commented=on  init=0  rst=off  en=off  dbl_ovrd=off  block_type=register
  Register2 : xbsIndex_r4/Register  Commented=on  init=0  rst=off  en=off  dbl_ovrd=off  block_type=register
  Relational : xbsIndex_r4/Relational  Commented=on  mode=a<b  op_type=Bool  en=off  latency=0  dbl_ovrd=off  block_type=relational
  State : Subsystem  Commented=on
  TwoPower : Subsystem  Commented=on
  TwoPower1 : Subsystem
  en : Outport
  k : Outport  Port=2
  n : Outport  Port=3
  wires:
  ? -> TwoPower/1(X)
  ? -> Register2/1, TwoPower/2(En)
  TwoPower/1(Y) -> Counter1/2, Relational/2
  ? -> NegEdgeDet/1(In1), State/2(Set)
  Counter1/1 -> Relational/1
  Relational/1 -> State/1(Clr), Counter1/4, Logical/1
  State/1(Out1) -> Logical/2
  Logical/1 -> ?
  Register2/1 -> Register1/1
  Register1/1 -> Counter1/1
  NegEdgeDet/1(Out1) -> Counter1/3
  nfft/1 -> TwoPower1/1(In)
  nfftWe/1 -> TwoPower1/2(En)
  start/1 -> MCode/1
  MCode/2 -> en/1
  TwoPower1/1(Out1) -> n/1, MCode/2
  MCode/1 -> k/1

== system hbf_fft/strobe ==
  In1 : Inport
  Inverter : xbsIndex_r4/Inverter  en=off  latency=0  dbl_ovrd=off  block_type=inv
  Logical : xbsIndex_r4/Logical  logical_function=AND  inputs=2  en=off  latency=0  precision=Full  arith_type=Unsigned  n_bits=16  bin_pt=0  align_bp=on  dbl_ovrd=off  block_type=logical
  Register : xbsIndex_r4/Register  init=0  rst=off  en=off  dbl_ovrd=off  block_type=register
  Register3 : xbsIndex_r4/Register  init=0  rst=off  en=off  dbl_ovrd=off  block_type=register
  Register4 : xbsIndex_r4/Register  init=0  rst=off  en=off  dbl_ovrd=off  block_type=register
  Out1 : Outport
  wires:
  In1/1 -> Register3/1
  Register/1 -> Logical/1
  Inverter/1 -> Logical/2
  Logical/1 -> Out1/1
  Register4/1 -> Inverter/1, Register/1
  Register3/1 -> Register4/1

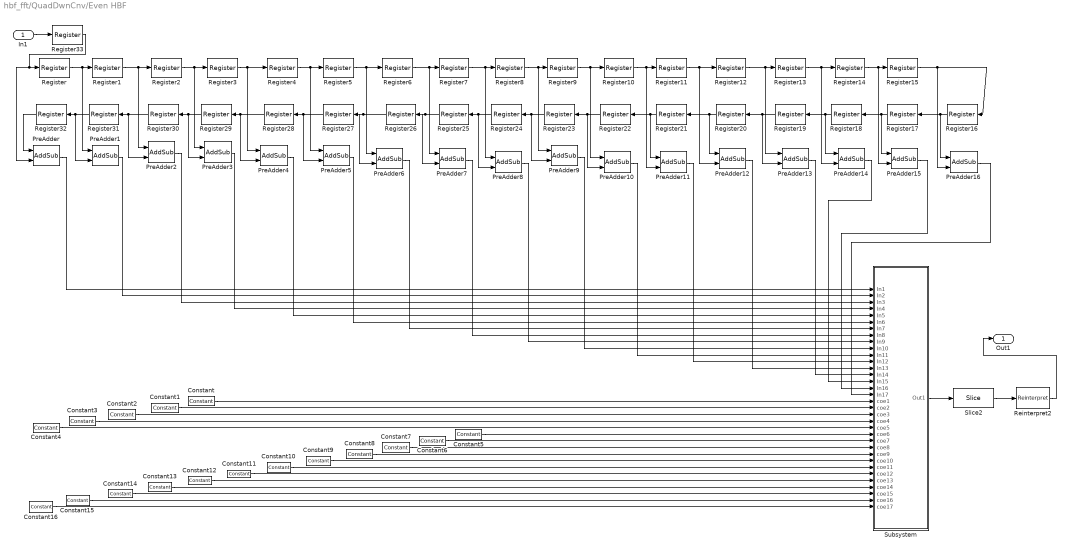
== system hbf_fft/QuadDwnCnv/Even HBF ==
  In1 : Inport
  Constant : xbsIndex_r4/Constant  const=coe(1)  gui_display_data_type=Fixed-point  arith_type=Signed (2's comp)  n_bits=numbits  bin_pt=binarypoint  preci_type=Single  exp_width=8  frac_width=24  explicit_period=off  period=1  equ=P=C  opselect=C  inp2=PCIN>>17  opr=+  inp1=P  carry=CIN  dbl_ovrd=off  block_type=constant
  Constant1 : xbsIndex_r4/Constant  const=coe(2)  gui_display_data_type=Fixed-point  arith_type=Signed (2's comp)  n_bits=numbits  bin_pt=binarypoint  preci_type=Single  exp_width=8  frac_width=24  explicit_period=off  period=1  equ=P=C  opselect=C  inp2=PCIN>>17  opr=+  inp1=P  carry=CIN  dbl_ovrd=off  block_type=constant
  Constant10 : xbsIndex_r4/Constant  const=coe(11)  gui_display_data_type=Fixed-point  arith_type=Signed (2's comp)  n_bits=numbits  bin_pt=binarypoint  preci_type=Single  exp_width=8  frac_width=24  explicit_period=off  period=1  equ=P=C  opselect=C  inp2=PCIN>>17  opr=+  inp1=P  carry=CIN  dbl_ovrd=off  block_type=constant
  Constant11 : xbsIndex_r4/Constant  const=coe(12)  gui_display_data_type=Fixed-point  arith_type=Signed (2's comp)  n_bits=numbits  bin_pt=binarypoint  preci_type=Single  exp_width=8  frac_width=24  explicit_period=off  period=1  equ=P=C  opselect=C  inp2=PCIN>>17  opr=+  inp1=P  carry=CIN  dbl_ovrd=off  block_type=constant
  Constant12 : xbsIndex_r4/Constant  const=coe(13)  gui_display_data_type=Fixed-point  arith_type=Signed (2's comp)  n_bits=numbits  bin_pt=binarypoint  preci_type=Single  exp_width=8  frac_width=24  explicit_period=off  period=1  equ=P=C  opselect=C  inp2=PCIN>>17  opr=+  inp1=P  carry=CIN  dbl_ovrd=off  block_type=constant
  Constant13 : xbsIndex_r4/Constant  const=coe(14)  gui_display_data_type=Fixed-point  arith_type=Signed (2's comp)  n_bits=numbits  bin_pt=binarypoint  preci_type=Single  exp_width=8  frac_width=24  explicit_period=off  period=1  equ=P=C  opselect=C  inp2=PCIN>>17  opr=+  inp1=P  carry=CIN  dbl_ovrd=off  block_type=constant
  Constant14 : xbsIndex_r4/Constant  const=coe(15)  gui_display_data_type=Fixed-point  arith_type=Signed (2's comp)  n_bits=numbits  bin_pt=binarypoint  preci_type=Single  exp_width=8  frac_width=24  explicit_period=off  period=1  equ=P=C  opselect=C  inp2=PCIN>>17  opr=+  inp1=P  carry=CIN  dbl_ovrd=off  block_type=constant
  Constant15 : xbsIndex_r4/Constant  const=coe(16)  gui_display_data_type=Fixed-point  arith_type=Signed (2's comp)  n_bits=numbits  bin_pt=binarypoint  preci_type=Single  exp_width=8  frac_width=24  explicit_period=off  period=1  equ=P=C  opselect=C  inp2=PCIN>>17  opr=+  inp1=P  carry=CIN  dbl_ovrd=off  block_type=constant
  Constant16 : xbsIndex_r4/Constant  const=coe(17)  gui_display_data_type=Fixed-point  arith_type=Signed (2's comp)  n_bits=numbits  bin_pt=binarypoint  preci_type=Single  exp_width=8  frac_width=24  explicit_period=off  period=1  equ=P=C  opselect=C  inp2=PCIN>>17  opr=+  inp1=P  carry=CIN  dbl_ovrd=off  block_type=constant
  Constant2 : xbsIndex_r4/Constant  const=coe(3)  gui_display_data_type=Fixed-point  arith_type=Signed (2's comp)  n_bits=numbits  bin_pt=binarypoint  preci_type=Single  exp_width=8  frac_width=24  explicit_period=off  period=1  equ=P=C  opselect=C  inp2=PCIN>>17  opr=+  inp1=P  carry=CIN  dbl_ovrd=off  block_type=constant
  Constant3 : xbsIndex_r4/Constant  const=coe(4)  gui_display_data_type=Fixed-point  arith_type=Signed (2's comp)  n_bits=numbits  bin_pt=binarypoint  preci_type=Single  exp_width=8  frac_width=24  explicit_period=off  period=1  equ=P=C  opselect=C  inp2=PCIN>>17  opr=+  inp1=P  carry=CIN  dbl_ovrd=off  block_type=constant
  Constant4 : xbsIndex_r4/Constant  const=coe(5)  gui_display_data_type=Fixed-point  arith_type=Signed (2's comp)  n_bits=numbits  bin_pt=binarypoint  preci_type=Single  exp_width=8  frac_width=24  explicit_period=off  period=1  equ=P=C  opselect=C  inp2=PCIN>>17  opr=+  inp1=P  carry=CIN  dbl_ovrd=off  block_type=constant
  Constant5 : xbsIndex_r4/Constant  const=coe(6)  gui_display_data_type=Fixed-point  arith_type=Signed (2's comp)  n_bits=numbits  bin_pt=binarypoint  preci_type=Single  exp_width=8  frac_width=24  explicit_period=off  period=1  equ=P=C  opselect=C  inp2=PCIN>>17  opr=+  inp1=P  carry=CIN  dbl_ovrd=off  block_type=constant
  Constant6 : xbsIndex_r4/Constant  const=coe(7)  gui_display_data_type=Fixed-point  arith_type=Signed (2's comp)  n_bits=numbits  bin_pt=binarypoint  preci_type=Single  exp_width=8  frac_width=24  explicit_period=off  period=1  equ=P=C  opselect=C  inp2=PCIN>>17  opr=+  inp1=P  carry=CIN  dbl_ovrd=off  block_type=constant
  Constant7 : xbsIndex_r4/Constant  const=coe(8)  gui_display_data_type=Fixed-point  arith_type=Signed (2's comp)  n_bits=numbits  bin_pt=binarypoint  preci_type=Single  exp_width=8  frac_width=24  explicit_period=off  period=1  equ=P=C  opselect=C  inp2=PCIN>>17  opr=+  inp1=P  carry=CIN  dbl_ovrd=off  block_type=constant
  Constant8 : xbsIndex_r4/Constant  const=coe(9)  gui_display_data_type=Fixed-point  arith_type=Signed (2's comp)  n_bits=numbits  bin_pt=binarypoint  preci_type=Single  exp_width=8  frac_width=24  explicit_period=off  period=1  equ=P=C  opselect=C  inp2=PCIN>>17  opr=+  inp1=P  carry=CIN  dbl_ovrd=off  block_type=constant
  Constant9 : xbsIndex_r4/Constant  const=coe(10)  gui_display_data_type=Fixed-point  arith_type=Signed (2's comp)  n_bits=numbits  bin_pt=binarypoint  preci_type=Single  exp_width=8  frac_width=24  explicit_period=off  period=1  equ=P=C  opselect=C  inp2=PCIN>>17  opr=+  inp1=P  carry=CIN  dbl_ovrd=off  block_type=constant
  PreAdder{,1..16} (17 alike) : xbsIndex_r4/AddSub  mode=Addition  use_carryin=off  use_carryout=off  en=off  latency=0  precision=Full  arith_type=Unsigned  n_bits=16  bin_pt=14  quantization=Truncate  overflow=Wrap  use_behavioral_HDL=off  hw_selection=Fabric  pipelined=off  use_rpm=on  dbl_ovrd=off  block_type=addsub
      settings: block_version=10.1.3
  Register{,1..33} (34 alike) : xbsIndex_r4/Register  init=0  rst=off  en=off  dbl_ovrd=off  block_type=register
  Reinterpret2 : xbsIndex_r4/Reinterpret  force_arith_type=on  arith_type="Signed  (2's comp)"  force_bin_pt=on  bin_pt=AD_BP  block_type=reinterpret
      settings: block_version=11.1
  Slice2 : xbsIndex_r4/Slice  nbits=AD_W  boolean_output=off  mode=Two Bit Locations  bit1=0  base1=Binary Point of Input  bit0=-AD_W+1  base0=Binary Point of Input  dbl_ovrd=off  block_type=slice
      settings: block_version=11.1
  Subsystem : Subsystem
  Out1 : Outport
  wires:
  Register/1 -> Register1/1, PreAdder1/1
  Register1/1 -> Register2/1, PreAdder2/1
  Register2/1 -> Register3/1, PreAdder3/1
  Register3/1 -> Register4/1, PreAdder4/1
  Register4/1 -> Register5/1, PreAdder5/1
  Register5/1 -> Register6/1, PreAdder6/1
  Register6/1 -> Register7/1, PreAdder7/1
  Register7/1 -> Register8/1, PreAdder8/1
  Register8/1 -> Register9/1, PreAdder9/1
  Register9/1 -> Register10/1, PreAdder10/1
  Register10/1 -> Register11/1, PreAdder11/2
  Register11/1 -> Register12/1, PreAdder12/2
  Register12/1 -> Register13/1, PreAdder13/1
  Register13/1 -> Register14/1, PreAdder14/2
  Register14/1 -> Register15/1, PreAdder15/2
  Register15/1 -> Register16/1, PreAdder16/2
  Register17/1 -> Register18/1, PreAdder15/1
  Register18/1 -> Register19/1, PreAdder14/1
  Register19/1 -> Register20/1, PreAdder13/2
  Register20/1 -> Register21/1, PreAdder12/1
  Register21/1 -> Register22/1, PreAdder11/1
  Register22/1 -> Register23/1, PreAdder10/2
  Register23/1 -> Register24/1, PreAdder9/2
  Register24/1 -> Register25/1, PreAdder8/2
  Register25/1 -> PreAdder7/2, Register26/1
  Register26/1 -> Register27/1, PreAdder6/2
  Register27/1 -> Register28/1, PreAdder5/2
  Register28/1 -> Register29/1, PreAdder4/2
  Register29/1 -> Register30/1, PreAdder3/2
  Register30/1 -> Register31/1, PreAdder2/2
  Register31/1 -> Register32/1, PreAdder1/2
  Register16/1 -> Register17/1, PreAdder16/1
  PreAdder/1 -> Subsystem/1(In1)
  PreAdder1/1 -> Subsystem/2(In2)
  PreAdder2/1 -> Subsystem/3(In3)
  PreAdder3/1 -> Subsystem/4(In4)
  PreAdder4/1 -> Subsystem/5(In5)
  PreAdder5/1 -> Subsystem/6(In6)
  PreAdder6/1 -> Subsystem/7(In7)
  PreAdder7/1 -> Subsystem/8(In8)
  PreAdder8/1 -> Subsystem/9(In9)
  PreAdder9/1 -> Subsystem/10(In10)
  PreAdder10/1 -> Subsystem/11(In11)
  PreAdder11/1 -> Subsystem/12(In12)
  PreAdder12/1 -> Subsystem/13(In13)
  PreAdder13/1 -> Subsystem/14(In14)
  PreAdder14/1 -> Subsystem/15(In15)
  PreAdder15/1 -> Subsystem/16(In16)
  PreAdder16/1 -> Subsystem/17(In17)
  Constant/1 -> Subsystem/18(coe1)
  Constant1/1 -> Subsystem/19(coe2)
  Constant2/1 -> Subsystem/20(coe3)
  Constant3/1 -> Subsystem/21(coe4)
  Constant4/1 -> Subsystem/22(coe5)
  Constant5/1 -> Subsystem/23(coe6)
  Constant6/1 -> Subsystem/24(coe7)
  Constant7/1 -> Subsystem/25(coe8)
  Constant8/1 -> Subsystem/26(coe9)
  Constant9/1 -> Subsystem/27(coe10)
  Constant10/1 -> Subsystem/28(coe11)
  Constant11/1 -> Subsystem/29(coe12)
  Constant12/1 -> Subsystem/30(coe13)
  Constant13/1 -> Subsystem/31(coe14)
  Constant14/1 -> Subsystem/32(coe15)
  Constant15/1 -> Subsystem/33(coe16)
  Constant16/1 -> Subsystem/34(coe17)
  In1/1 -> Register33/1
  Register33/1 -> Register/1, PreAdder/2
  Register32/1 -> PreAdder/1
  Slice2/1 -> Reinterpret2/1
  Subsystem/1(Out1) -> Slice2/1
  Reinterpret2/1 -> Out1/1

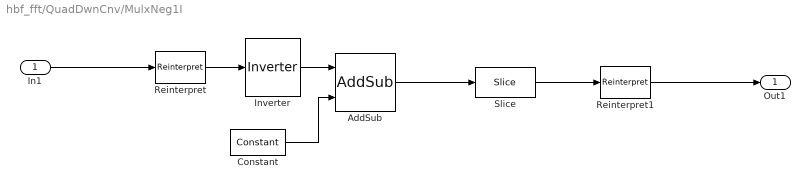
== system hbf_fft/QuadDwnCnv/MulxNeg1I ==
  In1 : Inport
  AddSub : xbsIndex_r4/AddSub  mode=Addition  use_carryin=off  use_carryout=off  en=off  latency=1  precision=Full  arith_type=Unsigned  n_bits=16  bin_pt=14  quantization=Truncate  overflow=Wrap  use_behavioral_HDL=off  hw_selection=Fabric  pipelined=off  dbl_ovrd=off  block_type=addsub
  Constant : xbsIndex_r4/Constant  const=1.0  gui_display_data_type=Fixed-point  arith_type=Unsigned  n_bits=1  bin_pt=0  preci_type=Single  exp_width=8  frac_width=24  explicit_period=off  period=1  equ=P=C  opselect=C  inp2=PCIN>>17  opr=+  inp1=P  carry=CIN  dbl_ovrd=off  block_type=constant
  Inverter : xbsIndex_r4/Inverter  en=off  latency=0  dbl_ovrd=off  block_type=inv
  Reinterpret : xbsIndex_r4/Reinterpret  force_arith_type=on  arith_type=Unsigned  force_bin_pt=on  bin_pt=0  block_type=reinterpret
  Reinterpret1 : xbsIndex_r4/Reinterpret  force_arith_type=on  arith_type="Signed  (2's comp)"  force_bin_pt=on  bin_pt=AD_BP  block_type=reinterpret
  Slice : xbsIndex_r4/Slice  nbits=16  boolean_output=off  mode=Two Bit Locations  bit1=-1  base1=MSB of Input  bit0=0  base0=LSB of Input  dbl_ovrd=off  block_type=slice
  Out1 : Outport
  wires:
  In1/1 -> Reinterpret/1
  Reinterpret1/1 -> Out1/1
  Inverter/1 -> AddSub/1
  Constant/1 -> AddSub/2
  Reinterpret/1 -> Inverter/1
  AddSub/1 -> Slice/1
  Slice/1 -> Reinterpret1/1

== system hbf_fft/QuadDwnCnv/MulxNeg1Q ==
  In1 : Inport
  AddSub : xbsIndex_r4/AddSub  mode=Addition  use_carryin=off  use_carryout=off  en=off  latency=1  precision=Full  arith_type=Unsigned  n_bits=16  bin_pt=14  quantization=Truncate  overflow=Wrap  use_behavioral_HDL=off  hw_selection=Fabric  pipelined=off  dbl_ovrd=off  block_type=addsub
  Constant : xbsIndex_r4/Constant  const=1.0  gui_display_data_type=Fixed-point  arith_type=Unsigned  n_bits=1  bin_pt=0  preci_type=Single  exp_width=8  frac_width=24  explicit_period=off  period=1  equ=P=C  opselect=C  inp2=PCIN>>17  opr=+  inp1=P  carry=CIN  dbl_ovrd=off  block_type=constant
  Inverter : xbsIndex_r4/Inverter  en=off  latency=0  dbl_ovrd=off  block_type=inv
  Reinterpret : xbsIndex_r4/Reinterpret  force_arith_type=on  arith_type=Unsigned  force_bin_pt=on  bin_pt=0  block_type=reinterpret
  Reinterpret1 : xbsIndex_r4/Reinterpret  force_arith_type=on  arith_type="Signed  (2's comp)"  force_bin_pt=on  bin_pt=AD_BP  block_type=reinterpret
  Slice : xbsIndex_r4/Slice  nbits=16  boolean_output=off  mode=Two Bit Locations  bit1=-1  base1=MSB of Input  bit0=0  base0=LSB of Input  dbl_ovrd=off  block_type=slice
  Out1 : Outport
  wires:
  In1/1 -> Reinterpret/1
  Reinterpret1/1 -> Out1/1
  Inverter/1 -> AddSub/1
  Constant/1 -> AddSub/2
  Reinterpret/1 -> Inverter/1
  AddSub/1 -> Slice/1
  Slice/1 -> Reinterpret1/1

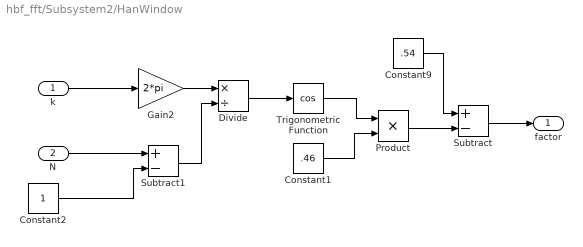
== system hbf_fft/Subsystem2/HanWindow ==
  k : Inport
  N : Inport  Port=2
  Constant1 : Constant  Value=.46
  Constant2 : Constant
  Constant9 : Constant  Value=.54
  Divide : Product  Inputs=*/
  Gain2 : Gain  Gain=2*pi
  Product : Product
  Subtract : Sum  Inputs=+-
  Subtract1 : Sum  Inputs=+-
  Trigonometric Function : Trigonometry  Operator=cos
  factor : Outport
  wires:
  Divide/1 -> Trigonometric Function/1
  Trigonometric Function/1 -> Product/1
  Product/1 -> Subtract/2
  k/1 -> Gain2/1
  Gain2/1 -> Divide/1
  N/1 -> Subtract1/1
  Constant2/1 -> Subtract1/2
  Subtract1/1 -> Divide/2
  Constant1/1 -> Product/2
  Constant9/1 -> Subtract/1
  Subtract/1 -> factor/1
